simulink model "lab7_t26"  (R2021a)
settings: Solver=VariableStepAuto  StartTime=0.0  StopTime=10.0  RelTol=1e-3
settings Model: Creator=reemb  LastModifiedBy=reemb

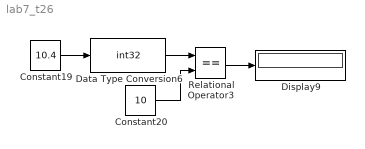
== system lab7_t26 ==
  Constant19 : Constant  Value=10.4
  Constant20 : Constant  Value=10
  Data Type Conversion6 : DataTypeConversion  OutDataTypeStr=int32  RndMeth=Round
  Display9 : Display
  Relational Operator3 : RelationalOperator  Operator===  OutDataTypeStr=boolean  RndMeth=Simplest
  wires:
  Data Type Conversion6/1 -> Relational Operator3/1
  Constant20/1 -> Relational Operator3/2
  Relational Operator3/1 -> Display9/1
  Constant19/1 -> Data Type Conversion6/1
